simulink model "ECSE308_Lab_2_2_1"  (R2019b)
settings: Solver=VariableStepAuto  StartTime=0.0  StopTime=10.0  RelTol=1e-3
libraries: commanabbnd3 x2, dspsrcs4 x1
settings Model: Creator=mikewang  LastModifiedBy=mikewang

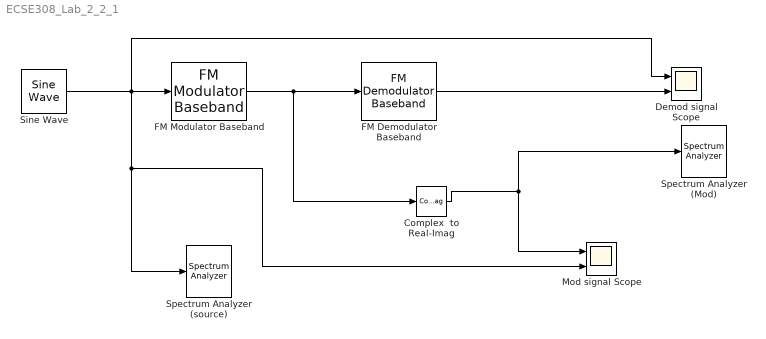
== system ECSE308_Lab_2_2_1 ==
  Complex  to Real-Imag : ComplexToRealImag  Output=Real
  Demod signal Scope : Scope  NumInputPorts=2
  "FM Demodulator Baseband " : commanabbnd3/FM Demodulator Baseband   FrequencyDeviation=50  SimulateUsing=Interpreted execution
      settings: SourceProductName=Communications Toolbox  SourceProductBaseCode=CM
  FM Modulator Baseband : commanabbnd3/FM Modulator Baseband  FrequencyDeviation=50  SimulateUsing=Interpreted execution
      settings: SourceProductName=Communications Toolbox  SourceProductBaseCode=CM
  Mod signal Scope : Scope  NumInputPorts=2
  "Sine Wave " : dspsrcs4/Sine Wave  Amplitude=1  Frequency=4  Phase=0  SampleMode=Discrete  OutComplex=Real  CompMethod=Trigonometric fcn  TableSize=Speed  SampleTime=1e-3  SamplesPerFrame=500  ResetState=Restart at time zero  OutputFrames=off  dataType=double  wordLen=16  udDataType=sfix(16)  fracBitsMode=Best precision  numFracBits=15  OutDataTypeStr=double  LastOutDataTypeStr=double
  Spectrum Analyzer (Mod) : SpectrumAnalyzer
  "Spectrum Analyzer (source) " : SpectrumAnalyzer
  wires:
  "FM Demodulator Baseband "/1 -> Demod signal Scope/2
  FM Modulator Baseband/1 -> Complex  to Real-Imag/1, "FM Demodulator Baseband "/1
  "Sine Wave "/1 -> Demod signal Scope/1, "Spectrum Analyzer (source) "/1, Mod signal Scope/2, FM Modulator Baseband/1
  Complex  to Real-Imag/1 -> Spectrum Analyzer (Mod)/1, Mod signal Scope/1
